simulink model "dsss"  (Simulink 7.1)
settings: Solver=ode45  StartTime=0.0  StopTime=0.80  RelTol=1e-3
libraries: simulink x264, dspbuff3 x24, dspxfrm3 x8, commsynccomp2 x5, dspsigops x4, dspobslib x4, dsparch4 x3, commutil2 x2, commseqgen2 x1, commfilt2 x1, commsink2 x1, dspspect3 x1
(part 4 of 4)

== system dsss/PN_DOPPLE/MF Subsystem/MF array/MF30 232-239/Subsystem ==
  In1 : Inport  OutDataType=sfix(16)  OutScaling=2^0
  Constant{12,14..17} (5 alike) : Constant  Value=-1  OutDataType=sfix(16)  OutScaling=2^0
  Constant13 : Constant  OutDataType=sfix(16)  OutScaling=2^0
  Constant18 : Constant  OutDataType=sfix(16)  OutScaling=2^0
  Constant9 : Constant  OutDataType=sfix(16)  OutScaling=2^0
  Integer Delay10 : simulink/Discrete/Integer Delay  vinit=0.0  samptime=-1  NumDelays=232
  Integer Delay13 : simulink/Discrete/Integer Delay  vinit=0.0  samptime=-1  NumDelays=236
  Integer Delay14 : simulink/Discrete/Integer Delay  vinit=0.0  samptime=-1  NumDelays=235
  Integer Delay15 : simulink/Discrete/Integer Delay  vinit=0.0  samptime=-1  NumDelays=234
  Integer Delay16 : simulink/Discrete/Integer Delay  vinit=0.0  samptime=-1  NumDelays=239
  Integer Delay17 : simulink/Discrete/Integer Delay  vinit=0.0  samptime=-1  NumDelays=238
  Integer Delay18 : simulink/Discrete/Integer Delay  vinit=0.0  samptime=-1  NumDelays=237
  Integer Delay9 : simulink/Discrete/Integer Delay  vinit=0.0  samptime=-1  NumDelays=233
  Product{9..10,13..18} (8 alike) : Product  OutDataType=sfix(16)  OutScaling=2^0  RndMeth=Zero
  Out1 : Outport  OutDataType=sfix(16)  OutScaling=2^0
  Out5 : Outport  Port=2  OutDataType=sfix(16)  OutScaling=2^0
  Out10 : Outport  Port=3  OutDataType=sfix(16)  OutScaling=2^0
  Out12 : Outport  Port=4  OutDataType=sfix(16)  OutScaling=2^0
  Out13 : Outport  Port=5  OutDataType=sfix(16)  OutScaling=2^0
  Out16 : Outport  Port=6  OutDataType=sfix(16)  OutScaling=2^0
  Out17 : Outport  Port=7  OutDataType=sfix(16)  OutScaling=2^0
  Out18 : Outport  Port=8  OutDataType=sfix(16)  OutScaling=2^0
  wires:
  Product10/1 -> Out16/1
  Product13/1 -> Out13/1
  Product9/1 -> Out12/1
  Product16/1 -> Out10/1
  Product15/1 -> Out5/1
  Product14/1 -> Out1/1
  Constant15/1 -> Product13/2
  Constant12/1 -> Product10/2
  Integer Delay15/1 -> Product14/1
  Constant13/1 -> Product14/2
  Integer Delay14/1 -> Product15/1
  Constant14/1 -> Product15/2
  Integer Delay13/1 -> Product16/1
  Constant16/1 -> Product16/2
  Integer Delay16/1 -> Product13/1
  Integer Delay10/1 -> Product9/1
  Constant9/1 -> Product9/2
  Integer Delay9/1 -> Product10/1
  In1/1 -> Integer Delay15/1, Integer Delay14/1, Integer Delay13/1, Integer Delay16/1, Integer Delay17/1, Integer Delay18/1, Integer Delay10/1, Integer Delay9/1
  Product17/1 -> Out17/1
  Constant17/1 -> Product17/2
  Integer Delay17/1 -> Product17/1
  Product18/1 -> Out18/1
  Constant18/1 -> Product18/2
  Integer Delay18/1 -> Product18/1

== system dsss/PN_DOPPLE/MF Subsystem/MF array/MF31 240-247/Subsystem ==
  In1 : Inport  OutDataType=sfix(16)  OutScaling=2^0
  Constant{1,3..4,8} (4 alike) : Constant  OutDataType=sfix(16)  OutScaling=2^0
  Constant{2,5..7} (4 alike) : Constant  Value=-1  OutDataType=sfix(16)  OutScaling=2^0
  Integer Delay1 : simulink/Discrete/Integer Delay  vinit=0.0  samptime=-1  NumDelays=243
  Integer Delay2 : simulink/Discrete/Integer Delay  vinit=0.0  samptime=-1  NumDelays=242
  Integer Delay3 : simulink/Discrete/Integer Delay  vinit=0.0  samptime=-1  NumDelays=241
  Integer Delay4 : simulink/Discrete/Integer Delay  vinit=0.0  samptime=-1  NumDelays=240
  Integer Delay5 : simulink/Discrete/Integer Delay  vinit=0.0  samptime=-1  NumDelays=247
  Integer Delay6 : simulink/Discrete/Integer Delay  vinit=0.0  samptime=-1  NumDelays=246
  Integer Delay7 : simulink/Discrete/Integer Delay  vinit=0.0  samptime=-1  NumDelays=245
  Integer Delay8 : simulink/Discrete/Integer Delay  vinit=0.0  samptime=-1  NumDelays=244
  Product{1..8} (8 alike) : Product  OutDataType=sfix(16)  OutScaling=2^0  RndMeth=Zero
  Out2 : Outport  OutDataType=sfix(16)  OutScaling=2^0
  Out3 : Outport  Port=2  OutDataType=sfix(16)  OutScaling=2^0
  Out6 : Outport  Port=3  OutDataType=sfix(16)  OutScaling=2^0
  Out7 : Outport  Port=4  OutDataType=sfix(16)  OutScaling=2^0
  Out9 : Outport  Port=5  OutDataType=sfix(16)  OutScaling=2^0
  Out11 : Outport  Port=6  OutDataType=sfix(16)  OutScaling=2^0
  Out14 : Outport  Port=7  OutDataType=sfix(16)  OutScaling=2^0
  Out15 : Outport  Port=8  OutDataType=sfix(16)  OutScaling=2^0
  wires:
  Integer Delay4/1 -> Product3/1
  Product6/1 -> Out15/1
  Product2/1 -> Out14/1
  Product5/1 -> Out11/1
  Product1/1 -> Out9/1
  Product8/1 -> Out7/1
  Product4/1 -> Out6/1
  Product7/1 -> Out3/1
  Product3/1 -> Out2/1
  Integer Delay8/1 -> Product7/1
  Constant6/1 -> Product7/2
  Integer Delay7/1 -> Product8/1
  Constant7/1 -> Product8/2
  Integer Delay6/1 -> Product5/1
  Constant5/1 -> Product5/2
  Integer Delay5/1 -> Product6/1
  Constant8/1 -> Product6/2
  Constant2/1 -> Product3/2
  Integer Delay3/1 -> Product4/1
  Constant3/1 -> Product4/2
  Integer Delay2/1 -> Product1/1
  Constant1/1 -> Product1/2
  Integer Delay1/1 -> Product2/1
  Constant4/1 -> Product2/2
  In1/1 -> Integer Delay4/1, Integer Delay1/1, Integer Delay2/1, Integer Delay3/1, Integer Delay8/1, Integer Delay7/1, Integer Delay6/1, Integer Delay5/1

== system dsss/PN_DOPPLE/MF Subsystem/MF array/MF32 248-255/Subsystem ==
  In1 : Inport  OutDataType=sfix(16)  OutScaling=2^0
  Constant{9..14,16} (7 alike) : Constant  Value=-1  OutDataType=sfix(16)  OutScaling=2^0
  Constant15 : Constant  OutDataType=sfix(16)  OutScaling=2^0
  Integer Delay10 : simulink/Discrete/Integer Delay  vinit=0.0  samptime=-1  NumDelays=250
  Integer Delay11 : simulink/Discrete/Integer Delay  vinit=0.0  samptime=-1  NumDelays=249
  Integer Delay12 : simulink/Discrete/Integer Delay  vinit=0.0  samptime=-1  NumDelays=248
  Integer Delay13 : simulink/Discrete/Integer Delay  vinit=0.0  samptime=-1  NumDelays=254
  Integer Delay14 : simulink/Discrete/Integer Delay  vinit=0.0  samptime=-1  NumDelays=253
  Integer Delay15 : simulink/Discrete/Integer Delay  vinit=0.0  samptime=-1  NumDelays=252
  Integer Delay16 : simulink/Discrete/Integer Delay  vinit=0.0  samptime=-1  NumDelays=255
  Integer Delay9 : simulink/Discrete/Integer Delay  vinit=0.0  samptime=-1  NumDelays=251
  Product{9..16} (8 alike) : Product  OutDataType=sfix(16)  OutScaling=2^0  RndMeth=Zero
  Out1 : Outport  OutDataType=sfix(16)  OutScaling=2^0
  Out4 : Outport  Port=2  OutDataType=sfix(16)  OutScaling=2^0
  Out5 : Outport  Port=3  OutDataType=sfix(16)  OutScaling=2^0
  Out8 : Outport  Port=4  OutDataType=sfix(16)  OutScaling=2^0
  Out10 : Outport  Port=5  OutDataType=sfix(16)  OutScaling=2^0
  Out12 : Outport  Port=6  OutDataType=sfix(16)  OutScaling=2^0
  Out13 : Outport  Port=7  OutDataType=sfix(16)  OutScaling=2^0
  Out16 : Outport  Port=8  OutDataType=sfix(16)  OutScaling=2^0
  wires:
  In1/1 -> Integer Delay16/1, Integer Delay13/1, Integer Delay14/1, Integer Delay15/1, Integer Delay9/1, Integer Delay10/1, Integer Delay11/1, Integer Delay12/1
  Integer Delay9/1 -> Product10/1
  Constant9/1 -> Product9/2
  Integer Delay10/1 -> Product9/1
  Constant11/1 -> Product12/2
  Integer Delay11/1 -> Product12/1
  Constant10/1 -> Product11/2
  Integer Delay12/1 -> Product11/1
  Integer Delay16/1 -> Product13/1
  Constant16/1 -> Product16/2
  Integer Delay13/1 -> Product16/1
  Constant14/1 -> Product15/2
  Integer Delay14/1 -> Product15/1
  Constant13/1 -> Product14/2
  Integer Delay15/1 -> Product14/1
  Constant12/1 -> Product10/2
  Constant15/1 -> Product13/2
  Product14/1 -> Out1/1
  Product11/1 -> Out4/1
  Product15/1 -> Out5/1
  Product12/1 -> Out8/1
  Product16/1 -> Out10/1
  Product9/1 -> Out12/1
  Product13/1 -> Out13/1
  Product10/1 -> Out16/1

== system dsss/PN_DOPPLE/MF Subsystem/MF array/MF4 24-31/Subsystem ==
  In1 : Inport  OutDataType=sfix(16)  OutScaling=2^0
  Constant10 : Constant  OutDataType=sfix(16)  OutScaling=2^0
  Constant{9,11,13..16} (6 alike) : Constant  Value=-1  OutDataType=sfix(16)  OutScaling=2^0
  Constant12 : Constant  OutDataType=sfix(16)  OutScaling=2^0
  Integer Delay10 : simulink/Discrete/Integer Delay  vinit=0.0  samptime=-1  NumDelays=26
  Integer Delay11 : simulink/Discrete/Integer Delay  vinit=0.0  samptime=-1  NumDelays=25
  Integer Delay12 : simulink/Discrete/Integer Delay  vinit=0.0  samptime=-1  NumDelays=24
  Integer Delay13 : simulink/Discrete/Integer Delay  vinit=0.0  samptime=-1  NumDelays=30
  Integer Delay14 : simulink/Discrete/Integer Delay  vinit=0.0  samptime=-1  NumDelays=29
  Integer Delay15 : simulink/Discrete/Integer Delay  vinit=0.0  samptime=-1  NumDelays=28
  Integer Delay16 : simulink/Discrete/Integer Delay  vinit=0.0  samptime=-1  NumDelays=31
  Integer Delay9 : simulink/Discrete/Integer Delay  vinit=0.0  samptime=-1  NumDelays=27
  Product{9..16} (8 alike) : Product  OutDataType=sfix(16)  OutScaling=2^0  RndMeth=Zero
  Out1 : Outport  OutDataType=sfix(16)  OutScaling=2^0
  Out2 : Outport  Port=2  OutDataType=sfix(16)  OutScaling=2^0
  Out3 : Outport  Port=3  OutDataType=sfix(16)  OutScaling=2^0
  Out4 : Outport  Port=4  OutDataType=sfix(16)  OutScaling=2^0
  Out5 : Outport  Port=5  OutDataType=sfix(16)  OutScaling=2^0
  Out6 : Outport  Port=6  OutDataType=sfix(16)  OutScaling=2^0
  Out7 : Outport  Port=7  OutDataType=sfix(16)  OutScaling=2^0
  Out8 : Outport  Port=8  OutDataType=sfix(16)  OutScaling=2^0
  wires:
  Product15/1 -> Out6/1
  Product10/1 -> Out4/1
  Product13/1 -> Out8/1
  Product9/1 -> Out3/1
  Product16/1 -> Out7/1
  Product12/1 -> Out2/1
  Product11/1 -> Out1/1
  Constant15/1 -> Product13/2
  Constant12/1 -> Product10/2
  Integer Delay15/1 -> Product14/1
  Constant13/1 -> Product14/2
  Integer Delay14/1 -> Product15/1
  Constant14/1 -> Product15/2
  Integer Delay13/1 -> Product16/1
  Constant16/1 -> Product16/2
  Integer Delay16/1 -> Product13/1
  Integer Delay12/1 -> Product11/1
  Constant10/1 -> Product11/2
  Integer Delay11/1 -> Product12/1
  Constant11/1 -> Product12/2
  Integer Delay10/1 -> Product9/1
  Constant9/1 -> Product9/2
  Integer Delay9/1 -> Product10/1
  In1/1 -> Integer Delay12/1, Integer Delay11/1, Integer Delay10/1, Integer Delay9/1, Integer Delay15/1, Integer Delay14/1, Integer Delay13/1, Integer Delay16/1
  Product14/1 -> Out5/1

== system dsss/PN_DOPPLE/MF Subsystem/MF array/MF5 32-39/Subsystem ==
  In1 : Inport  OutDataType=sfix(16)  OutScaling=2^0
  Constant{1,6,8,10..11} (5 alike) : Constant  OutDataType=sfix(16)  OutScaling=2^0
  Constant4 : Constant  Value=-1  OutDataType=sfix(16)  OutScaling=2^0
  Constant5 : Constant  Value=-1  OutDataType=sfix(16)  OutScaling=2^0
  Constant7 : Constant  Value=-1  OutDataType=sfix(16)  OutScaling=2^0
  Integer Delay1 : simulink/Discrete/Integer Delay  vinit=0.0  samptime=-1  NumDelays=33
  Integer Delay11 : simulink/Discrete/Integer Delay  vinit=0.0  samptime=-1  NumDelays=39
  Integer Delay12 : simulink/Discrete/Integer Delay  vinit=0.0  samptime=-1  NumDelays=38
  Integer Delay2 : simulink/Discrete/Integer Delay  vinit=0.0  samptime=-1  NumDelays=32
  Integer Delay5 : simulink/Discrete/Integer Delay  vinit=0.0  samptime=-1  NumDelays=37
  Integer Delay6 : simulink/Discrete/Integer Delay  vinit=0.0  samptime=-1  NumDelays=36
  Integer Delay7 : simulink/Discrete/Integer Delay  vinit=0.0  samptime=-1  NumDelays=35
  Integer Delay8 : simulink/Discrete/Integer Delay  vinit=0.0  samptime=-1  NumDelays=34
  Product{1..2,5..8,11..12} (8 alike) : Product  OutDataType=sfix(16)  OutScaling=2^0  RndMeth=Zero
  Out1 : Outport  OutDataType=sfix(16)  OutScaling=2^0
  Out2 : Outport  Port=2  OutDataType=sfix(16)  OutScaling=2^0
  Out3 : Outport  Port=3  OutDataType=sfix(16)  OutScaling=2^0
  Out4 : Outport  Port=4  OutDataType=sfix(16)  OutScaling=2^0
  Out5 : Outport  Port=5  OutDataType=sfix(16)  OutScaling=2^0
  Out6 : Outport  Port=6  OutDataType=sfix(16)  OutScaling=2^0
  Out7 : Outport  Port=7  OutDataType=sfix(16)  OutScaling=2^0
  Out8 : Outport  Port=8  OutDataType=sfix(16)  OutScaling=2^0
  wires:
  Product6/1 -> Out6/1
  Product2/1 -> Out2/1
  Product5/1 -> Out5/1
  Product1/1 -> Out1/1
  Integer Delay6/1 -> Product5/1
  Constant5/1 -> Product5/2
  Integer Delay5/1 -> Product6/1
  Constant8/1 -> Product6/2
  Integer Delay2/1 -> Product1/1
  Constant1/1 -> Product1/2
  Integer Delay1/1 -> Product2/1
  Constant4/1 -> Product2/2
  In1/1 -> Integer Delay2/1, Integer Delay1/1, Integer Delay8/1, Integer Delay7/1, Integer Delay6/1, Integer Delay5/1, Integer Delay12/1, Integer Delay11/1
  Product8/1 -> Out4/1
  Product7/1 -> Out3/1
  Integer Delay8/1 -> Product7/1
  Constant6/1 -> Product7/2
  Integer Delay7/1 -> Product8/1
  Constant7/1 -> Product8/2
  Product12/1 -> Out8/1
  Product11/1 -> Out7/1
  Integer Delay12/1 -> Product11/1
  Constant10/1 -> Product11/2
  Integer Delay11/1 -> Product12/1
  Constant11/1 -> Product12/2

== system dsss/PN_DOPPLE/MF Subsystem/MF array/MF6 40-47/Subsystem ==
  In1 : Inport  OutDataType=sfix(16)  OutScaling=2^0
  Constant{9,12,14..15,18} (5 alike) : Constant  OutDataType=sfix(16)  OutScaling=2^0
  Constant13 : Constant  Value=-1  OutDataType=sfix(16)  OutScaling=2^0
  Constant16 : Constant  Value=-1  OutDataType=sfix(16)  OutScaling=2^0
  Constant17 : Constant  Value=-1  OutDataType=sfix(16)  OutScaling=2^0
  Integer Delay10 : simulink/Discrete/Integer Delay  vinit=0.0  samptime=-1  NumDelays=40
  Integer Delay13 : simulink/Discrete/Integer Delay  vinit=0.0  samptime=-1  NumDelays=44
  Integer Delay14 : simulink/Discrete/Integer Delay  vinit=0.0  samptime=-1  NumDelays=43
  Integer Delay15 : simulink/Discrete/Integer Delay  vinit=0.0  samptime=-1  NumDelays=42
  Integer Delay16 : simulink/Discrete/Integer Delay  vinit=0.0  samptime=-1  NumDelays=45
  Integer Delay17 : simulink/Discrete/Integer Delay  vinit=0.0  samptime=-1  NumDelays=47
  Integer Delay18 : simulink/Discrete/Integer Delay  vinit=0.0  samptime=-1  NumDelays=46
  Integer Delay9 : simulink/Discrete/Integer Delay  vinit=0.0  samptime=-1  NumDelays=41
  Product{9..10,13..18} (8 alike) : Product  OutDataType=sfix(16)  OutScaling=2^0  RndMeth=Zero
  Out1 : Outport  OutDataType=sfix(16)  OutScaling=2^0
  Out2 : Outport  Port=2  OutDataType=sfix(16)  OutScaling=2^0
  Out3 : Outport  Port=3  OutDataType=sfix(16)  OutScaling=2^0
  Out4 : Outport  Port=4  OutDataType=sfix(16)  OutScaling=2^0
  Out5 : Outport  Port=5  OutDataType=sfix(16)  OutScaling=2^0
  Out6 : Outport  Port=6  OutDataType=sfix(16)  OutScaling=2^0
  Out7 : Outport  Port=7  OutDataType=sfix(16)  OutScaling=2^0
  Out8 : Outport  Port=8  OutDataType=sfix(16)  OutScaling=2^0
  wires:
  In1/1 -> Integer Delay10/1, Integer Delay9/1, Integer Delay15/1, Integer Delay14/1, Integer Delay13/1, Integer Delay16/1, Integer Delay18/1, Integer Delay17/1
  Integer Delay9/1 -> Product10/1
  Constant9/1 -> Product9/2
  Integer Delay10/1 -> Product9/1
  Integer Delay16/1 -> Product13/1
  Constant16/1 -> Product16/2
  Integer Delay13/1 -> Product16/1
  Constant12/1 -> Product10/2
  Constant15/1 -> Product13/2
  Constant17/1 -> Product17/2
  Integer Delay17/1 -> Product18/1
  Constant18/1 -> Product18/2
  Integer Delay18/1 -> Product17/1
  Constant14/1 -> Product15/2
  Integer Delay14/1 -> Product15/1
  Constant13/1 -> Product14/2
  Integer Delay15/1 -> Product14/1
  Product9/1 -> Out1/1
  Product10/1 -> Out2/1
  Product14/1 -> Out3/1
  Product15/1 -> Out4/1
  Product16/1 -> Out5/1
  Product13/1 -> Out6/1
  Product17/1 -> Out7/1
  Product18/1 -> Out8/1

== system dsss/PN_DOPPLE/MF Subsystem/MF array/MF7 48-55/Subsystem ==
  In1 : Inport  OutDataType=sfix(16)  OutScaling=2^0
  Constant{1,5,8,10..11} (5 alike) : Constant  Value=-1  OutDataType=sfix(16)  OutScaling=2^0
  Constant4 : Constant  OutDataType=sfix(16)  OutScaling=2^0
  Constant6 : Constant  OutDataType=sfix(16)  OutScaling=2^0
  Constant7 : Constant  OutDataType=sfix(16)  OutScaling=2^0
  Integer Delay1 : simulink/Discrete/Integer Delay  vinit=0.0  samptime=-1  NumDelays=49
  Integer Delay11 : simulink/Discrete/Integer Delay  vinit=0.0  samptime=-1  NumDelays=55
  Integer Delay12 : simulink/Discrete/Integer Delay  vinit=0.0  samptime=-1  NumDelays=54
  Integer Delay2 : simulink/Discrete/Integer Delay  vinit=0.0  samptime=-1  NumDelays=48
  Integer Delay5 : simulink/Discrete/Integer Delay  vinit=0.0  samptime=-1  NumDelays=53
  Integer Delay6 : simulink/Discrete/Integer Delay  vinit=0.0  samptime=-1  NumDelays=52
  Integer Delay7 : simulink/Discrete/Integer Delay  vinit=0.0  samptime=-1  NumDelays=51
  Integer Delay8 : simulink/Discrete/Integer Delay  vinit=0.0  samptime=-1  NumDelays=50
  Product{1..2,5..8,11..12} (8 alike) : Product  OutDataType=sfix(16)  OutScaling=2^0  RndMeth=Zero
  Out1 : Outport  OutDataType=sfix(16)  OutScaling=2^0
  Out2 : Outport  Port=2  OutDataType=sfix(16)  OutScaling=2^0
  Out3 : Outport  Port=3  OutDataType=sfix(16)  OutScaling=2^0
  Out4 : Outport  Port=4  OutDataType=sfix(16)  OutScaling=2^0
  Out5 : Outport  Port=5  OutDataType=sfix(16)  OutScaling=2^0
  Out6 : Outport  Port=6  OutDataType=sfix(16)  OutScaling=2^0
  Out7 : Outport  Port=7  OutDataType=sfix(16)  OutScaling=2^0
  Out8 : Outport  Port=8  OutDataType=sfix(16)  OutScaling=2^0
  wires:
  In1/1 -> Integer Delay2/1, Integer Delay1/1, Integer Delay5/1, Integer Delay6/1, Integer Delay7/1, Integer Delay8/1, Integer Delay12/1, Integer Delay11/1
  Constant4/1 -> Product2/2
  Integer Delay1/1 -> Product2/1
  Constant1/1 -> Product1/2
  Integer Delay2/1 -> Product1/1
  Constant8/1 -> Product6/2
  Integer Delay5/1 -> Product6/1
  Constant5/1 -> Product5/2
  Integer Delay6/1 -> Product5/1
  Constant7/1 -> Product8/2
  Integer Delay7/1 -> Product8/1
  Constant6/1 -> Product7/2
  Integer Delay8/1 -> Product7/1
  Constant11/1 -> Product12/2
  Integer Delay11/1 -> Product12/1
  Constant10/1 -> Product11/2
  Integer Delay12/1 -> Product11/1
  Product7/1 -> Out3/1
  Product11/1 -> Out7/1
  Product8/1 -> Out4/1
  Product12/1 -> Out8/1
  Product1/1 -> Out1/1
  Product5/1 -> Out5/1
  Product2/1 -> Out2/1
  Product6/1 -> Out6/1

== system dsss/PN_DOPPLE/MF Subsystem/MF array/MF8 55-62/Subsystem ==
  In1 : Inport  OutDataType=sfix(16)  OutScaling=2^0
  Constant12 : Constant  OutDataType=sfix(16)  OutScaling=2^0
  Constant13 : Constant  OutDataType=sfix(16)  OutScaling=2^0
  Constant{9,14..16,18} (5 alike) : Constant  Value=-1  OutDataType=sfix(16)  OutScaling=2^0
  Constant17 : Constant  OutDataType=sfix(16)  OutScaling=2^0
  Integer Delay10 : simulink/Discrete/Integer Delay  vinit=0.0  samptime=-1  NumDelays=56
  Integer Delay13 : simulink/Discrete/Integer Delay  vinit=0.0  samptime=-1  NumDelays=60
  Integer Delay14 : simulink/Discrete/Integer Delay  vinit=0.0  samptime=-1  NumDelays=59
  Integer Delay15 : simulink/Discrete/Integer Delay  vinit=0.0  samptime=-1  NumDelays=58
  Integer Delay16 : simulink/Discrete/Integer Delay  vinit=0.0  samptime=-1  NumDelays=61
  Integer Delay17 : simulink/Discrete/Integer Delay  vinit=0.0  samptime=-1  NumDelays=63
  Integer Delay18 : simulink/Discrete/Integer Delay  vinit=0.0  samptime=-1  NumDelays=62
  Integer Delay9 : simulink/Discrete/Integer Delay  vinit=0.0  samptime=-1  NumDelays=57
  Product{9..10,13..18} (8 alike) : Product  OutDataType=sfix(16)  OutScaling=2^0  RndMeth=Zero
  Out1 : Outport  OutDataType=sfix(16)  OutScaling=2^0
  Out2 : Outport  Port=2  OutDataType=sfix(16)  OutScaling=2^0
  Out3 : Outport  Port=3  OutDataType=sfix(16)  OutScaling=2^0
  Out4 : Outport  Port=4  OutDataType=sfix(16)  OutScaling=2^0
  Out5 : Outport  Port=5  OutDataType=sfix(16)  OutScaling=2^0
  Out6 : Outport  Port=6  OutDataType=sfix(16)  OutScaling=2^0
  Out7 : Outport  Port=7  OutDataType=sfix(16)  OutScaling=2^0
  Out8 : Outport  Port=8  OutDataType=sfix(16)  OutScaling=2^0
  wires:
  Product10/1 -> Out2/1
  Product13/1 -> Out6/1
  Product16/1 -> Out5/1
  Product15/1 -> Out4/1
  Constant15/1 -> Product13/2
  Constant12/1 -> Product10/2
  Integer Delay15/1 -> Product14/1
  Constant13/1 -> Product14/2
  Integer Delay14/1 -> Product15/1
  Constant14/1 -> Product15/2
  Integer Delay13/1 -> Product16/1
  Constant16/1 -> Product16/2
  Integer Delay16/1 -> Product13/1
  Integer Delay10/1 -> Product9/1
  Constant9/1 -> Product9/2
  Integer Delay9/1 -> Product10/1
  In1/1 -> Integer Delay15/1, Integer Delay14/1, Integer Delay13/1, Integer Delay16/1, Integer Delay18/1, Integer Delay17/1, Integer Delay10/1, Integer Delay9/1
  Constant18/1 -> Product18/2
  Integer Delay17/1 -> Product18/1
  Constant17/1 -> Product17/2
  Product17/1 -> Out7/1
  Product18/1 -> Out8/1
  Integer Delay18/1 -> Product17/1
  Product9/1 -> Out1/1
  Product14/1 -> Out3/1

== system dsss/PN_DOPPLE/MF Subsystem/MF array/MF9 64-71/Subsystem ==
  In1 : Inport  OutDataType=sfix(16)  OutScaling=2^0
  Constant{1,6..7,10..11} (5 alike) : Constant  OutDataType=sfix(16)  OutScaling=2^0
  Constant4 : Constant  Value=-1  OutDataType=sfix(16)  OutScaling=2^0
  Constant5 : Constant  Value=-1  OutDataType=sfix(16)  OutScaling=2^0
  Constant8 : Constant  Value=-1  OutDataType=sfix(16)  OutScaling=2^0
  Integer Delay1 : simulink/Discrete/Integer Delay  vinit=0.0  samptime=-1  NumDelays=65
  Integer Delay11 : simulink/Discrete/Integer Delay  vinit=0.0  samptime=-1  NumDelays=71
  Integer Delay12 : simulink/Discrete/Integer Delay  vinit=0.0  samptime=-1  NumDelays=70
  Integer Delay2 : simulink/Discrete/Integer Delay  vinit=0.0  samptime=-1  NumDelays=64
  Integer Delay5 : simulink/Discrete/Integer Delay  vinit=0.0  samptime=-1  NumDelays=69
  Integer Delay6 : simulink/Discrete/Integer Delay  vinit=0.0  samptime=-1  NumDelays=68
  Integer Delay7 : simulink/Discrete/Integer Delay  vinit=0.0  samptime=-1  NumDelays=67
  Integer Delay8 : simulink/Discrete/Integer Delay  vinit=0.0  samptime=-1  NumDelays=66
  Product{1..2,5..8,11..12} (8 alike) : Product  OutDataType=sfix(16)  OutScaling=2^0  RndMeth=Zero
  Out1 : Outport  OutDataType=sfix(16)  OutScaling=2^0
  Out2 : Outport  Port=2  OutDataType=sfix(16)  OutScaling=2^0
  Out3 : Outport  Port=3  OutDataType=sfix(16)  OutScaling=2^0
  Out4 : Outport  Port=4  OutDataType=sfix(16)  OutScaling=2^0
  Out5 : Outport  Port=5  OutDataType=sfix(16)  OutScaling=2^0
  Out6 : Outport  Port=6  OutDataType=sfix(16)  OutScaling=2^0
  Out7 : Outport  Port=7  OutDataType=sfix(16)  OutScaling=2^0
  Out8 : Outport  Port=8  OutDataType=sfix(16)  OutScaling=2^0
  wires:
  Product6/1 -> Out6/1
  Product2/1 -> Out2/1
  Product5/1 -> Out5/1
  Product1/1 -> Out1/1
  Product12/1 -> Out8/1
  Product8/1 -> Out4/1
  Product11/1 -> Out7/1
  Product7/1 -> Out3/1
  Integer Delay12/1 -> Product11/1
  Constant10/1 -> Product11/2
  Integer Delay11/1 -> Product12/1
  Constant11/1 -> Product12/2
  Integer Delay8/1 -> Product7/1
  Constant6/1 -> Product7/2
  Integer Delay7/1 -> Product8/1
  Constant7/1 -> Product8/2
  Integer Delay6/1 -> Product5/1
  Constant5/1 -> Product5/2
  Integer Delay5/1 -> Product6/1
  Constant8/1 -> Product6/2
  Integer Delay2/1 -> Product1/1
  Constant1/1 -> Product1/2
  Integer Delay1/1 -> Product2/1
  Constant4/1 -> Product2/2
  In1/1 -> Integer Delay1/1, Integer Delay2/1, Integer Delay8/1, Integer Delay7/1, Integer Delay6/1, Integer Delay5/1, Integer Delay12/1, Integer Delay11/1

== system dsss/PN_DOPPLE/Local PN/local PN sequence Include Track/Local System/[1 0 0 1 1 1 0 1]PN/Enabled Subsystem ==
  In1 : Inport  OutDataType=sfix(16)  OutScaling=2^0
  Enable : EnablePort
  Unit Delay : UnitDelay  X0=1  SampleTime=-1
  Out1 : Outport  OutDataType=sfix(16)  OutScaling=2^0
  wires:
  In1/1 -> Unit Delay/1
  Unit Delay/1 -> Out1/1

== system dsss/PN_DOPPLE/Local PN/local PN sequence Include Track/Local System/[1 0 0 1 1 1 0 1]PN/Enabled Subsystem1 ==
  In1 : Inport  OutDataType=sfix(16)  OutScaling=2^0
  Enable : EnablePort
  Unit Delay : UnitDelay  SampleTime=-1
  Out1 : Outport  OutDataType=sfix(16)  OutScaling=2^0
  wires:
  Unit Delay/1 -> Out1/1
  In1/1 -> Unit Delay/1

== system dsss/PN_DOPPLE/Local PN/local PN sequence Include Track/Local System/[1 0 0 1 1 1 0 1]PN/Enabled Subsystem2 ==
  In1 : Inport  OutDataType=sfix(16)  OutScaling=2^0
  Enable : EnablePort
  Unit Delay : UnitDelay  SampleTime=-1
  Out1 : Outport  OutDataType=sfix(16)  OutScaling=2^0
  wires:
  In1/1 -> Unit Delay/1
  Unit Delay/1 -> Out1/1

== system dsss/PN_DOPPLE/Local PN/local PN sequence Include Track/Local System/[1 0 0 1 1 1 0 1]PN/Enabled Subsystem3 ==
  In1 : Inport  OutDataType=sfix(16)  OutScaling=2^0
  Enable : EnablePort
  Unit Delay : UnitDelay  SampleTime=-1
  Out1 : Outport  OutDataType=sfix(16)  OutScaling=2^0
  wires:
  Unit Delay/1 -> Out1/1
  In1/1 -> Unit Delay/1

== system dsss/PN_DOPPLE/Local PN/local PN sequence Include Track/Local System/[1 0 0 1 1 1 0 1]PN/Enabled Subsystem4 ==
  In1 : Inport  OutDataType=sfix(16)  OutScaling=2^0
  Enable : EnablePort
  Unit Delay : UnitDelay  SampleTime=-1
  Out1 : Outport  OutDataType=sfix(16)  OutScaling=2^0
  wires:
  In1/1 -> Unit Delay/1
  Unit Delay/1 -> Out1/1

== system dsss/PN_DOPPLE/Local PN/local PN sequence Include Track/Local System/[1 0 0 1 1 1 0 1]PN/Enabled Subsystem5 ==
  In1 : Inport  OutDataType=sfix(16)  OutScaling=2^0
  Enable : EnablePort
  Unit Delay : UnitDelay  SampleTime=-1
  Out1 : Outport  OutDataType=sfix(16)  OutScaling=2^0
  wires:
  Unit Delay/1 -> Out1/1
  In1/1 -> Unit Delay/1

== system dsss/PN_DOPPLE/Local PN/local PN sequence Include Track/Local System/[1 0 0 1 1 1 0 1]PN/Enabled Subsystem6 ==
  In1 : Inport  OutDataType=sfix(16)  OutScaling=2^0
  Enable : EnablePort
  Unit Delay : UnitDelay  SampleTime=-1
  Out1 : Outport  OutDataType=sfix(16)  OutScaling=2^0
  wires:
  In1/1 -> Unit Delay/1
  Unit Delay/1 -> Out1/1

== system dsss/PN_DOPPLE/Local PN/local PN sequence Include Track/Local System/[1 0 0 1 1 1 0 1]PN/Enabled Subsystem7 ==
  In1 : Inport  OutDataType=sfix(16)  OutScaling=2^0
  Enable : EnablePort
  Unit Delay : UnitDelay  SampleTime=-1
  Out1 : Outport  OutDataType=sfix(16)  OutScaling=2^0
  wires:
  Unit Delay/1 -> Out1/1
  In1/1 -> Unit Delay/1
